simulink model "BDamperOk"  (R2018b)
settings: Solver=FixedStepDiscrete  StartTime=0.0  StopTime=10.0  FixedStep=0.001  RelTol=1e-3  SampleTimeConstraint=STIndependent
undefined symbols (not defined in the file): VDamperErrorHigh, VDamperErrorLow
libraries: simulink x8
settings Model: DataDictionary=Master_Dictionary.sldd  Creator=torni  LastModifiedBy=rubyg
settings RTWCC: SystemTargetFile=irt.tlc  TemplateMakefile=irt_default_tmf  Description=INTECRIO Real-Time Target
settings STFCustomTargetCC: TargetLangStandard=C99 (ISO)  UtilityFuncGeneration=Shared location  CombineOutputUpdateFcns=on  SystemTargetFile=irt.tlc
settings GRTTargetCC: UtilityFuncGeneration=Shared location  ParMdlRefBuildCompliant=off  CompOptLevelCompliant=off  ConcurrentExecutionCompliant=off  MatFileLogging=off  CPPClassGenCompliant=off  UseToolchainInfoCompliant=off  GenerateASAP2=on

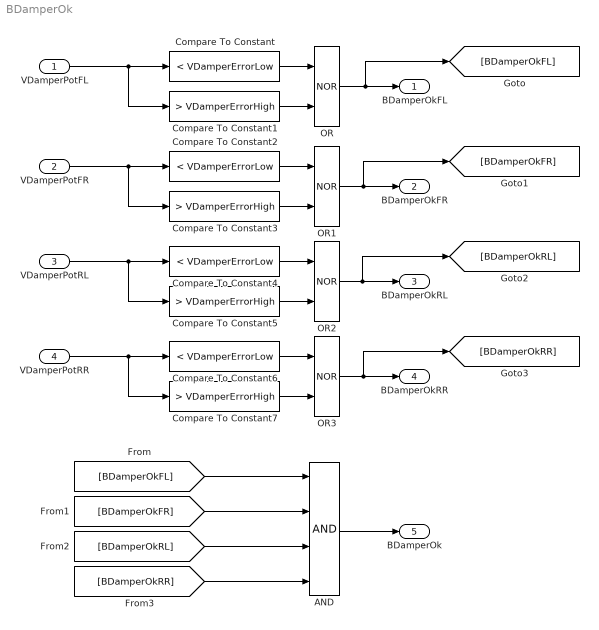
== system BDamperOk ==
  VDamperPotFL : Inport  OutDataTypeStr=double
  "VDamperPotFR " : Inport  Port=2  OutDataTypeStr=double
  VDamperPotRL : Inport  Port=3  OutDataTypeStr=double
  VDamperPotRR : Inport  Port=4  OutDataTypeStr=double
  AND : Logic  Inputs=4  AllPortsSameDT=off  OutDataTypeStr=boolean
  Compare To Constant{,2,4,6} (4 alike) : simulink/Logic and Bit Operations/Compare To Constant  relop=<  const=VDamperErrorLow  OutDataTypeStr=boolean
  Compare To Constant{1,3,5,7} (4 alike) : simulink/Logic and Bit Operations/Compare To Constant  relop=>  const=VDamperErrorHigh  OutDataTypeStr=boolean
  OR{,1..3} (4 alike) : Logic  Operator=NOR  AllPortsSameDT=off  OutDataTypeStr=boolean
  BDamperOkFL : Outport  OutDataTypeStr=boolean
  BDamperOkFR : Outport  Port=2  OutDataTypeStr=boolean
  BDamperOkRL : Outport  Port=3  OutDataTypeStr=boolean
  BDamperOkRR : Outport  Port=4  OutDataTypeStr=boolean
  BDamperOk : Outport  Port=5  OutDataTypeStr=boolean
  wires:
  Compare To Constant1/1 -> OR/2
  Compare To Constant/1 -> OR/1
  OR3/1 -> [BDamperOkRR], BDamperOkRR/1
  VDamperPotFL/1 -> Compare To Constant1/1, Compare To Constant/1
  OR/1 -> [BDamperOkFL], BDamperOkFL/1
  OR1/1 -> [BDamperOkFR], BDamperOkFR/1
  "VDamperPotFR "/1 -> Compare To Constant2/1, Compare To Constant3/1
  Compare To Constant2/1 -> OR1/1
  Compare To Constant3/1 -> OR1/2
  Compare To Constant5/1 -> OR2/2
  Compare To Constant4/1 -> OR2/1
  VDamperPotRL/1 -> Compare To Constant5/1, Compare To Constant4/1
  OR2/1 -> [BDamperOkRL], BDamperOkRL/1
  VDamperPotRR/1 -> Compare To Constant6/1, Compare To Constant7/1
  Compare To Constant6/1 -> OR3/1
  Compare To Constant7/1 -> OR3/2
  [BDamperOkRR] -> AND/4
  [BDamperOkRL] -> AND/3
  [BDamperOkFR] -> AND/2
  [BDamperOkFL] -> AND/1
  AND/1 -> BDamperOk/1
